simulink model "jili_mode_test"  (R2018b)
settings: Solver=VariableStepAuto  StartTime=0.0  StopTime=80  RelTol=1e-3
settings Model: Creator=erange  LastModifiedBy=erange

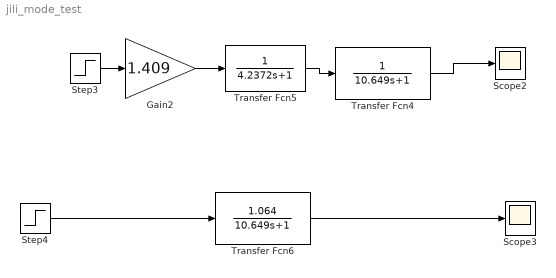
== system jili_mode_test ==
  Gain2 : Gain  Gain=1.409
  Scope2 : Scope
  Scope3 : Scope
  Step3 : Step  Time=0  SampleTime=0
  Step4 : Step  Time=0  After=-1  SampleTime=0
  Transfer Fcn4 : TransferFcn  Denominator=[10.649 1]
  Transfer Fcn5 : TransferFcn  Denominator=[4.2372 1]
  Transfer Fcn6 : TransferFcn  Numerator=[1.064]  Denominator=[10.649 1]
  wires:
  Transfer Fcn5/1 -> Transfer Fcn4/1
  Gain2/1 -> Transfer Fcn5/1
  Step4/1 -> Transfer Fcn6/1
  Transfer Fcn4/1 -> Scope2/1
  Step3/1 -> Gain2/1
  Transfer Fcn6/1 -> Scope3/1
